simulink model "rtwdemo_tflmatops"  (Simulink 7.6)
settings: Solver=FixedStepDiscrete  StartTime=0.0  StopTime=20  FixedStep=.01  RelTol=1e-3  SampleTimeConstraint=Specified
PreLoadFcn:
  | addpath(fullfile(matlabroot,'toolbox','rtw','rtwdemos','tfl_demo'));
  | sl_refresh_customizations;
libraries: rtwdemowidgets x2
settings Model: Creator=The MathWorks Inc.  ExtModeAutoUpdateStatusClock=off
settings MATStruct: SampleTime=1  Offset=0  Priority=[30.0]
settings DataIOCC: SaveOutput=off  SaveTime=off  SignalLoggingName=sigsOut
settings OptimizationCC: InlineParams=on  InlineInvariantSignals=on  PassReuseOutputArgsAs=Individual arguments  StateBitsets=on  DataBitsets=on  UseTempVars=on  ZeroExternalMemoryAtStartup=off  ZeroInternalMemoryAtStartup=off  NoFixptDivByZeroProtection=on  EfficientFloat2IntCast=on  EfficientMapNaN2IntZero=off  OptimizeModelRefInitCode=on  LifeSpan=1
settings DebuggingCC: CheckExecutionContextPreStartOutputMsg=on  CheckExecutionContextRuntimeOutputMsg=on  SolverPrmCheckMsg=none  IntegerOverflowMsg=none  StrictBusMsg=ErrorOnBusTreatedAsVector
settings HardwareCC: ProdIntDivRoundTo=Zero  ProdEndianess=LittleEndian  ProdHWDeviceType=Generic->32-bit Embedded Processor  TargetHWDeviceType=32-bit Generic
settings SFSimCC: SFSimEnableDebug=off  SFSimOverflowDetection=off  SimParseCustomCode=off
settings RTWCC: SystemTargetFile=ert.tlc  TemplateMakefile=ert_default_tmf  Description=Real-Time Workshop Embedded Coder (no auto configuration)  GenerateReport=on  RTWVerbose=off  ProcessScript=ert_make_rtw_hook  IncludeHyperlinkInReport=on  LaunchReport=on
settings CodeAppCC: ForceParamTrailComments=on  IgnoreCustomStorageClasses=off  IgnoreTestpoints=on  SimulinkDataObjDesc=on  CustomSymbolStrGlobalVar=rt$N$M  CustomSymbolStrType=$N$M  CustomSymbolStrFcn=$N$M$F  CustomSymbolStrMacro=$N$M  InsertBlockDesc=on
settings ERTTargetCC: TargetFunctionLibrary=Matrix Operation Examples  MultiwordLength=2048  GenerateSampleERTMain=on  IncludeMdlTerminateFcn=off  SupportAbsoluteTime=off  SupportNonFinite=off  InlinedParameterPlacement=NonHierarchical  ERTCustomFileTemplate=example_file_process.tlc  ConvertIfToSwitch=off

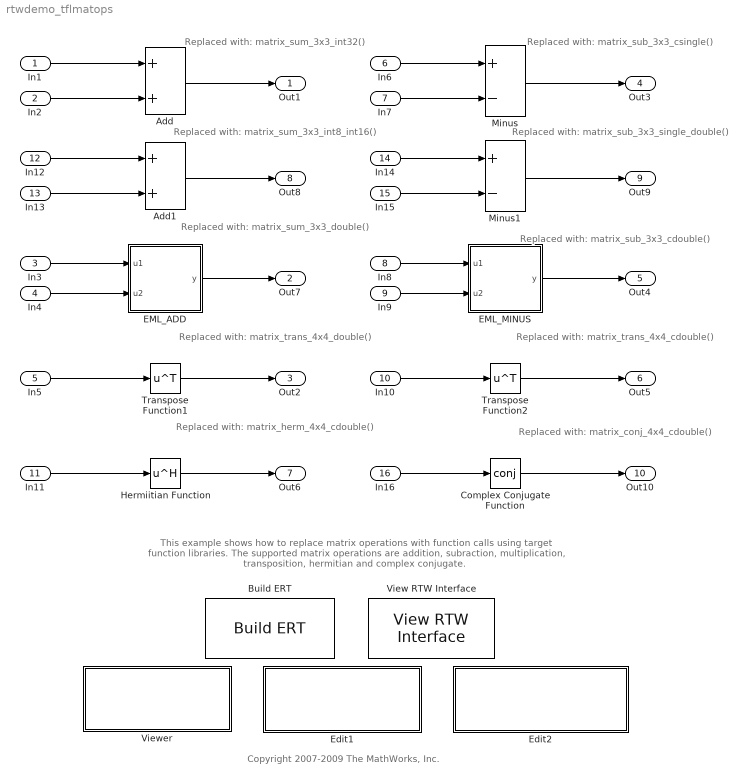
== system rtwdemo_tflmatops ==
  note: Copyright 2007-2009 The MathWorks, Inc.
  note: Replaced with:
      | matrix_sum_3x3_int32()
  note: Replaced with:
      | matrix_sum_3x3_double()
  note: Replaced with:
      | matrix_trans_4x4_double()
  note: Replaced with:
      | matrix_sub_3x3_csingle()
  note: Replaced with:
      | matrix_sub_3x3_cdouble()
  note: Replaced with:
      | matrix_trans_4x4_cdouble()
  note: This example shows how to replace matrix operations with
      | function calls using target function libraries.
      |
      | The supported matrix operations are addition, subraction, multiplication, transposition, hermitian and  complex conjugate.
  note: Replaced with:
      | matrix_herm_4x4_cdouble()
  note: Replaced with:
      | matrix_sum_3x3_int8_int16()
  note: Replaced with:
      | matrix_sub_3x3_single_double()
  note: Replaced with:
      | matrix_conj_4x4_cdouble()
  In1 : Inport  OutDataTypeStr=int32  PortDimensions=[3 3]  SampleTime=1
  In2 : Inport  Port=2  OutDataTypeStr=int32  PortDimensions=[3 3]  SampleTime=1
  In3 : Inport  Port=3  OutDataTypeStr=double  PortDimensions=[3 3]  SampleTime=1
  In4 : Inport  Port=4  OutDataTypeStr=double  PortDimensions=[3 3]  SampleTime=1
  In5 : Inport  Port=5  OutDataTypeStr=double  PortDimensions=[4 4]  SampleTime=1
  In6 : Inport  Port=6  OutDataTypeStr=single  PortDimensions=[3 3]  SampleTime=1
      settings: SignalType=complex
  In7 : Inport  Port=7  OutDataTypeStr=single  PortDimensions=[3 3]  SampleTime=1
      settings: SignalType=complex
  In8 : Inport  Port=8  OutDataTypeStr=double  PortDimensions=[3 3]  SampleTime=1
      settings: SignalType=complex
  In9 : Inport  Port=9  OutDataTypeStr=double  PortDimensions=[3 3]  SampleTime=1
      settings: SignalType=complex
  In10 : Inport  Port=10  OutDataTypeStr=double  PortDimensions=[4 4]  SampleTime=1
      settings: SignalType=complex
  In11 : Inport  Port=11  OutDataTypeStr=double  PortDimensions=[4 4]  SampleTime=1
      settings: SignalType=complex
  In12 : Inport  Port=12  OutDataTypeStr=int8  PortDimensions=[3 3]  SampleTime=1
  In13 : Inport  Port=13  OutDataTypeStr=int16  PortDimensions=[3 3]  SampleTime=1
  In14 : Inport  Port=14  OutDataTypeStr=single  PortDimensions=[3 3]  SampleTime=1
  In15 : Inport  Port=15  OutDataTypeStr=double  PortDimensions=[3 3]  SampleTime=1
  In16 : Inport  Port=16  OutDataTypeStr=double  PortDimensions=[4 4]  SampleTime=1
      settings: SignalType=complex
  Add : Sum  SaturateOnIntegerOverflow=on
  Add1 : Sum  SaturateOnIntegerOverflow=on
  Build ERT : rtwdemowidgets/Build ERT  SystemSampleTime=-1  attrib_overrides={'GenFloatMathFcnCalls', 'SupportComplex'}
  Complex Conjugate Function : Math  Operator=conj  SaturateOnIntegerOverflow=on
  EML_ADD : Stateflow chart  TreatAsAtomicUnit=on
  EML_MINUS : Stateflow chart  TreatAsAtomicUnit=on
  Edit1 : Subsystem  mask{attrib_overrides={}}
      mask prompts: attrib_overrides "List of attributes to preserve (cell of strings):"
      mask help: Enter the attributes of the configuration set that you want preserved. Otherwise, the default configuration script will override your current settings.
      settings: OpenFcn=edit('tfl_table_matrixop');
      mask Display:
      | disp(['View/edit TFL Definition\n',...
      | 	  'tfl_table_matrixop.m\n(double-click)'])
  Edit2 : Subsystem  mask{attrib_overrides={}}
      mask prompts: attrib_overrides "List of attributes to preserve (cell of strings):"
      mask help: Enter the attributes of the configuration set that you want preserved. Otherwise, the default configuration script will override your current settings.
      settings: OpenFcn=edit(fullfile(matlabroot,'toolbox','rtw','rtwdemos','tfl_demo', 'sl_customization.m'));
      mask Display:
      | disp(['View/edit TFL Registration\n',...
      | 	  'sl_customization.m\n(double-click)'])
  Hermiitian Function : Math  Operator=hermitian  SaturateOnIntegerOverflow=on
  Minus : Sum  Inputs=+-  SaturateOnIntegerOverflow=on
  Minus1 : Sum  Inputs=+-  SaturateOnIntegerOverflow=on
  Transpose Function1 : Math  Operator=transpose  SaturateOnIntegerOverflow=on
  Transpose Function2 : Math  Operator=transpose  SaturateOnIntegerOverflow=on
  View RTW Interface : rtwdemowidgets/View RTW Interface  SystemSampleTime=-1
  Viewer : Subsystem  mask{attrib_overrides={}}
      mask prompts: attrib_overrides "List of attributes to preserve (cell of strings):"
      mask help: Enter the attributes of the configuration set that you want preserved. Otherwise, the default configuration script will override your current settings.
      settings: OpenFcn=|
      | tfl = tfl_table_matrixop;
      | obj = RTW.viewTfl(tfl);
      | clear tfl obj;
      mask Display:
      | disp(['Invoke TFL Viewer on\n',...
      | 	  'tfl_table_matrixops.m\n(double-click)'])
  Out1 : Outport
  Out7 : Outport  Port=2
  Out2 : Outport  Port=3
  Out3 : Outport  Port=4
  Out4 : Outport  Port=5
  Out5 : Outport  Port=6
  Out6 : Outport  Port=7
  Out8 : Outport  Port=8
  Out9 : Outport  Port=9
  Out10 : Outport  Port=10
  wires:
  Add/1 -> Out1/1
  In1/1 -> Add/1
  In2/1 -> Add/2
  EML_ADD/1(y) -> Out7/1
  Transpose Function1/1 -> Out2/1
  Minus/1 -> Out3/1
  EML_MINUS/1(y) -> Out4/1
  Transpose Function2/1 -> Out5/1
  In3/1 -> EML_ADD/1(u1)
  In4/1 -> EML_ADD/2(u2)
  In5/1 -> Transpose Function1/1
  In6/1 -> Minus/1
  In7/1 -> Minus/2
  In8/1 -> EML_MINUS/1(u1)
  In9/1 -> EML_MINUS/2(u2)
  In10/1 -> Transpose Function2/1
  Hermiitian Function/1 -> Out6/1
  In11/1 -> Hermiitian Function/1
  Add1/1 -> Out8/1
  In12/1 -> Add1/1
  In13/1 -> Add1/2
  Minus1/1 -> Out9/1
  In14/1 -> Minus1/1
  In15/1 -> Minus1/2
  Complex Conjugate Function/1 -> Out10/1
  In16/1 -> Complex Conjugate Function/1

== system rtwdemo_tflmatops/Edit1 ==

== system rtwdemo_tflmatops/Edit2 ==

== system rtwdemo_tflmatops/Viewer ==

== matlab function EML_MINUS ==
  data: u1 input uint32; y output uint32; u2 input uint32
function y = fcn(u1, u2)
% This block supports the Embedded MATLAB subset.
% See the help menu for details. 

y = u1 - u2;

== matlab function EML_ADD ==
  data: u1 input uint32; y output uint32; u2 input uint32
function y = fcn(u1, u2)
% This block supports the Embedded MATLAB subset.
% See the help menu for details. 

y = u1 + u2;
